simulink model "Direct"  (R2015b)
settings: Solver=VariableStepAuto  StartTime=0.0  StopTime=10.0  RelTol=1e-3
values from neighbouring files (symbols this model uses):
  f = 50    [DirectControl2.m]
  L = XL/(2*2*pi*f)    (= 0.159154943092)    [DirectControl2.m]
  Sbase = 1000e6/2    (= 500000000)    [DirectControl2.m]
  Ts = 5e-6    (= 5e-06)    [DirectControl2.m]
  Tsample = 5e-4    (= 0.0005)    [DirectControl2.m]
  Vdc = 5    [DirectControl2.m]
  Vr = 220e3    (= 220000)    [DirectControl2.m]
  Vs = 220e3    (= 220000)    [DirectControl2.m]
undefined symbols (not defined in the file or in its folder): Ki, Kp
libraries: powerlib_meascontrol x32, powerlib x28, simulink x2, simulink_extras x1
settings Model: Creator=Sourabh Suri  LastModifiedBy=Sourabh Suri

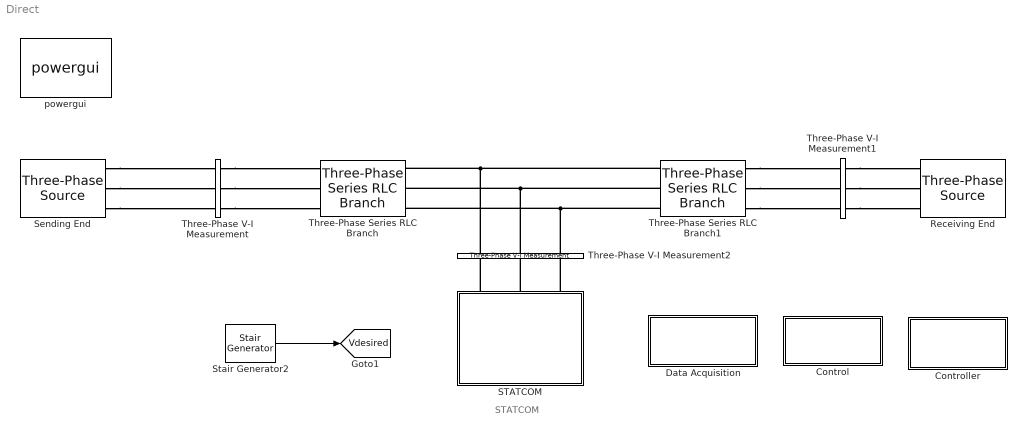
== system Direct ==
  note: STATCOM
  Control : Subsystem
  Controller : Subsystem
  Data Acquisition : Subsystem
  Receiving End : powerlib/Electrical Sources/Three-Phase Source  InternalConnection=Yg  VoltagePhases=off  Voltage=Vr  PhaseAngle=dr  Voltage_phases=[25e3 25e3 25e3]/sqrt(3)  PhaseAngles_phases=[0 -120 +120]  Frequency=f  NonIdealSource=off  SpecifyImpedance=off  Resistance=0.8929  Inductance=16.58e-3  ShortCircuitLevel=100e6  BaseVoltage=25e3  XRratio=7  BusType=swing  Pref=10e3  Qref=0  Prefabc=[10e3, 10e3, 10e3]  Qrefabc=[0, 0, 0]  Qmin=-inf  Qmax=inf
  STATCOM : Subsystem
  Sending End : powerlib/Electrical Sources/Three-Phase Source  InternalConnection=Yg  VoltagePhases=off  Voltage=Vs  PhaseAngle=ds  Voltage_phases=[25e3 25e3 25e3]/sqrt(3)  PhaseAngles_phases=[0 -120 +120]  Frequency=f  NonIdealSource=off  SpecifyImpedance=off  Resistance=0  Inductance=0  ShortCircuitLevel=100e6  BaseVoltage=0  XRratio=7  BusType=swing  Pref=10e3  Qref=0  Prefabc=[10e3, 10e3, 10e3]  Qrefabc=[0, 0, 0]  Qmin=-inf  Qmax=inf
  Stair Generator2 : powerlib_meascontrol/Pulse & Signal Generators/Stair Generator  t=[0 1 2 3 4 5 6 7]  e=[ 0.07 0.08 0.09 0.1 0.11 0.12 0.13 0.07]  Ts=Ts
  Three-Phase Series RLC Branch : powerlib/Elements/Three-Phase Series RLC Branch  LConnTagsString=A|B|C  RConnTagsString=A|B|C  BranchType=L  Resistance=1  Inductance=L  Capacitance=1e-6  Measurements=None
  Three-Phase Series RLC Branch1 : powerlib/Elements/Three-Phase Series RLC Branch  LConnTagsString=A|B|C  RConnTagsString=A|B|C  BranchType=L  Resistance=1  Inductance=L  Capacitance=1e-6  Measurements=None
  Three-Phase V-I Measurement : powerlib/Measurements/Three-Phase V-I Measurement  VoltageMeasurement=phase-to-phase  SetLabelV=on  LabelV=Vsabc  Vpu=off  VpuLL=on  CurrentMeasurement=yes  SetLabelI=on  LabelI=Isabc  Ipu=on  Pbase=Sbase  Vbase=Vn  OutputType=Complex  PhasorSimulation=off  PSBequivalent=0
  Three-Phase V-I Measurement1 : powerlib/Measurements/Three-Phase V-I Measurement  VoltageMeasurement=phase-to-phase  SetLabelV=on  LabelV=Vrabc  Vpu=off  VpuLL=on  CurrentMeasurement=yes  SetLabelI=on  LabelI=Irabc  Ipu=on  Pbase=Sbase  Vbase=Vn  OutputType=Complex  PhasorSimulation=off  PSBequivalent=0
  Three-Phase V-I Measurement2 : powerlib/Measurements/Three-Phase V-I Measurement  VoltageMeasurement=phase-to-phase  SetLabelV=on  LabelV=Vmabc  Vpu=off  VpuLL=on  CurrentMeasurement=yes  SetLabelI=on  LabelI=Imabc  Ipu=on  Pbase=Sbase  Vbase=Vn  OutputType=Complex  PhasorSimulation=off  PSBequivalent=0
  powergui : powerlib/powergui  Priority=1  SimulationMode=Discrete  SolverType=Backward Euler  SampleTime=Ts  frequency=60  SPID=on  DisableSnubberDevices=on  DisableRonSwitches=on  DisableVfSwitches=on  SwTol=0  DisplayEquations=off  Interpol=off  ExternalGateDelay=off  methode=off  Ts=10  FunctionMessages=off  echomessages=off  HookPort=off  EnableUseOfTLC=off  x0status=blocks  frequencyindice=50  Pbase=100e6  ErrMax=1e-4  Iterations=50  UnitsV=kV  UnitsW=MW  buscounter=0  RestoreLinks=warning  ResistiveCurrentMeasurement=off  Frange=[0:2:500]  Ylog=off  Xlog=on  ShowGrid=off  save=off  variable=ZData  structure=0  ZoomFFT=off  StartTime=0.0  cycles=1  DisplayStyle=1  fundamental=60  FreqAxis=off  MaxFrequency=1000  frequencyindicesteady=1  RmsSteady=1  display=off
  tag scope: Vdesired=global
  wires:
  Stair Generator2/1 -> [Vdesired]
  connections:
  Three-Phase V-I Measurement2/RConn1 -- Three-Phase Series RLC Branch/RConn1 -- Three-Phase Series RLC Branch1/RConn1
  Three-Phase V-I Measurement2/RConn2 -- Three-Phase Series RLC Branch/RConn2 -- Three-Phase Series RLC Branch1/RConn2
  Three-Phase V-I Measurement2/RConn3 -- Three-Phase Series RLC Branch/RConn3 -- Three-Phase Series RLC Branch1/RConn3
  Sending End/RConn1 -- Three-Phase V-I Measurement/LConn1
  Sending End/RConn2 -- Three-Phase V-I Measurement/LConn2
  Three-Phase V-I Measurement1/LConn2 -- Receiving End/RConn2
  Three-Phase V-I Measurement1/LConn1 -- Receiving End/RConn1
  Three-Phase Series RLC Branch1/LConn3 -- Three-Phase V-I Measurement1/RConn3
  Three-Phase V-I Measurement/RConn2 -- Three-Phase Series RLC Branch/LConn2
  Three-Phase V-I Measurement/RConn1 -- Three-Phase Series RLC Branch/LConn1
  Three-Phase V-I Measurement1/LConn3 -- Receiving End/RConn3
  Three-Phase V-I Measurement/RConn3 -- Three-Phase Series RLC Branch/LConn3
  Three-Phase Series RLC Branch1/LConn1 -- Three-Phase V-I Measurement1/RConn1
  Three-Phase Series RLC Branch1/LConn2 -- Three-Phase V-I Measurement1/RConn2
  Sending End/RConn3 -- Three-Phase V-I Measurement/LConn3
  STATCOM/LConn1 -- Three-Phase V-I Measurement2/LConn1
  STATCOM/LConn2 -- Three-Phase V-I Measurement2/LConn2
  STATCOM/LConn3 -- Three-Phase V-I Measurement2/LConn3

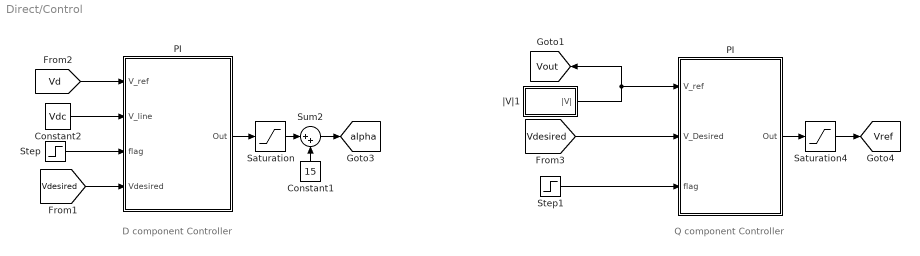
== system Direct/Control ==
  note: Q component Controller
  note: D component Controller
  Constant1 : Constant  Value=15
  Constant2 : Constant  Value=Vdc
  PI : MATLAB Function  TreatAsAtomicUnit=on
  "PI " : MATLAB Function  TreatAsAtomicUnit=on
  Saturation : Saturate  UpperLimit=45  LowerLimit=-25
  Saturation4 : Saturate  UpperLimit=1/sqrt(3)  LowerLimit=0.057
  Step : Step  Time=0.1  SampleTime=0
  Step1 : Step  Time=.04  SampleTime=0
  Sum2 : Sum  Inputs=|++  SaturateOnIntegerOverflow=on  InputSameDT=on  OutDataTypeStr=Inherit: Same as first input
  |V|1 : Subsystem
  tag scope: Vout=global, Vref=global, alpha=global
  wires:
  [Vd] -> PI/1(V_ref)
  PI/1(Out) -> Saturation/1
  Constant1/1 -> Sum2/2
  Step/1 -> PI/3(flag)
  Constant2/1 -> PI/2(V_line)
  |V|1/1(|V|) -> "PI "/1(V_ref), [Vout]
  "PI "/1(Out) -> Saturation4/1
  [Vdesired] -> "PI "/2(V_Desired)
  Step1/1 -> "PI "/3(flag)
  Saturation4/1 -> [Vref]
  Saturation/1 -> Sum2/1
  [Vdesired] -> PI/4(Vdesired)
  Sum2/1 -> [alpha]

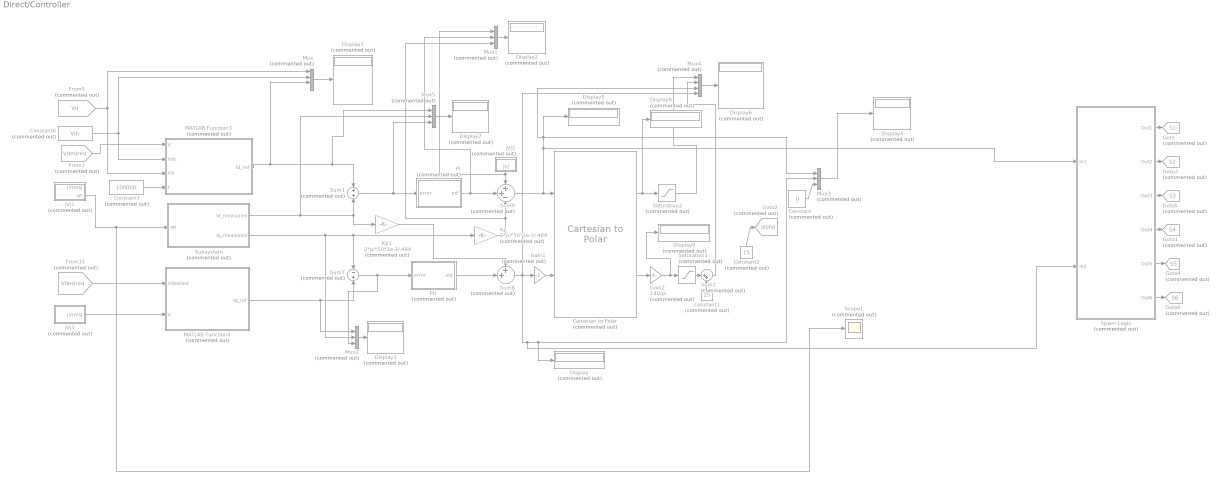
== system Direct/Controller ==
  Cartesian to Polar : simulink_extras/Transformations/Cartesian to Polar  Commented=on
  Constant : Constant  Commented=on  Value=0
  Constant1 : Constant  Commented=on  Value=15
  Constant2 : Constant  Commented=on  Value=15
  Constant3 : Constant  Commented=on  Value=100000
  Constant6 : Constant  Commented=on  Value=Vdc
  Display{,1..9} (10 alike) : Display  Commented=on
  From1 : From  Commented=on  GotoTag=Vdesired  TagVisibility=global
  From11 : From  Commented=on  GotoTag=Vdesired  TagVisibility=global
  From5 : From  Commented=on  GotoTag=Vd  TagVisibility=global
  Gain1 : Gain  Commented=on  Gain=-1
  Gain2 : Gain  Commented=on  Gain=180/pi
  Goto : Goto  Commented=on  GotoTag=S1  TagVisibility=global
  Goto1 : Goto  Commented=on  GotoTag=S4  TagVisibility=global
  Goto2 : Goto  Commented=on  GotoTag=alpha  TagVisibility=global
  Goto3 : Goto  Commented=on  GotoTag=S2  TagVisibility=global
  Goto4 : Goto  Commented=on  GotoTag=S5  TagVisibility=global
  Goto5 : Goto  Commented=on  GotoTag=S3  TagVisibility=global
  Goto6 : Goto  Commented=on  GotoTag=S6  TagVisibility=global
  Kp : Gain  Commented=on  Gain=2*pi*50*1e-3/.484
  Kp1 : Gain  Commented=on  Gain=2*pi*50*1e-3/.484
  MATLAB Function3 : MATLAB Function  Commented=on  TreatAsAtomicUnit=on
  MATLAB Function4 : MATLAB Function  Commented=on  TreatAsAtomicUnit=on
  Mux : Mux  Commented=on
  Mux{1..3,5} (4 alike) : Mux  Commented=on  Inputs=3
  Mux4 : Mux  Commented=on
  PI : Subsystem  Commented=on
  PI1 : Subsystem  Commented=on
  Saturation1 : Saturate  Commented=on  UpperLimit=2  LowerLimit=-28.5  LinearizeAsGain=off  ZeroCross=off
  Saturation2 : Saturate  Commented=on  UpperLimit=Vdc/sqrt(3)  LowerLimit=Vdc*.1e-9
  Scope1 : Scope  Commented=on
  Spwm Logic : Subsystem  Commented=on
  Subsystem : Subsystem  Commented=on
  Sum1 : Sum  Commented=on
  Sum2 : Sum  Commented=on  Inputs=|++  SaturateOnIntegerOverflow=on  InputSameDT=on  OutDataTypeStr=Inherit: Same as first input
  Sum7 : Sum  Commented=on  Inputs=-+
  Sum8 : Sum  Commented=on  Inputs=++|
  Sum9 : Sum  Commented=on  Inputs=++-
  |V|1 : Subsystem  Commented=on
  |V|2 : Subsystem  Commented=on
  |V|3 : Subsystem  Commented=on
  wires:
  Constant6/1 -> MATLAB Function3/2(Vdc), Mux/2
  From5/1 -> MATLAB Function3/3(Vd), Mux/1
  Mux/1 -> Display1/1
  |V|2/1(|V|) -> Mux1/1, Sum9/1
  Subsystem/2(Iq_measured) -> Mux2/2, Kp/1, Sum7/1
  Kp/1 -> Mux1/3, Sum9/3
  From11/1 -> MATLAB Function4/1(Vdesired)
  |V|3/1(|Vrms|) -> MATLAB Function4/2(V)
  Sum7/1 -> Mux2/3, PI1/1(error)
  PI1/1(eq') -> Sum8/2
  Kp1/1 -> Sum8/1
  Mux4/1 -> Display6/1
  Subsystem/1(Id_measured) -> Mux5/2, Kp1/1, Sum1/2
  MATLAB Function3/1(Id_ref) -> Mux5/1, Sum1/1, Mux/3
  Mux5/1 -> Display7/1
  Sum1/1 -> Mux5/3, PI/1(error)
  Cartesian to Polar/1 -> Display8/1, Saturation2/1
  Mux1/1 -> Display2/1
  PI/1(ed') -> Mux1/2, Sum9/2
  Mux2/1 -> Display3/1
  MATLAB Function4/1(Iq_ref) -> Mux2/1, Sum7/2
  Mux3/1 -> Display4/1
  |V|1/2(wt) -> Scope1/1, Subsystem/1(wt)
  Constant/1 -> Mux3/3
  Saturation1/1 -> Sum2/1
  Constant1/1 -> Sum2/2
  Sum8/1 -> Spwm Logic/2(In2), Display/1, Mux3/2, Gain1/1, Mux4/4
  Sum2/1 -> Mux4/2
  Saturation2/1 -> Mux4/1
  Cartesian to Polar/2 -> Gain2/1
  Gain1/1 -> Cartesian to Polar/2
  Sum9/1 -> Mux4/3, Mux3/1, Display5/1, Spwm Logic/1(In1), Cartesian to Polar/1
  Constant2/1 -> Goto2/1
  Spwm Logic/2(Out2) -> Goto3/1
  Spwm Logic/1(Out1) -> Goto/1
  Spwm Logic/3(Out3) -> Goto5/1
  Spwm Logic/4(Out4) -> Goto1/1
  Spwm Logic/5(Out5) -> Goto4/1
  Spwm Logic/6(Out6) -> Goto6/1
  Constant3/1 -> MATLAB Function3/4(t)
  From1/1 -> MATLAB Function3/1(V)
  Gain2/1 -> Display9/1, Saturation1/1

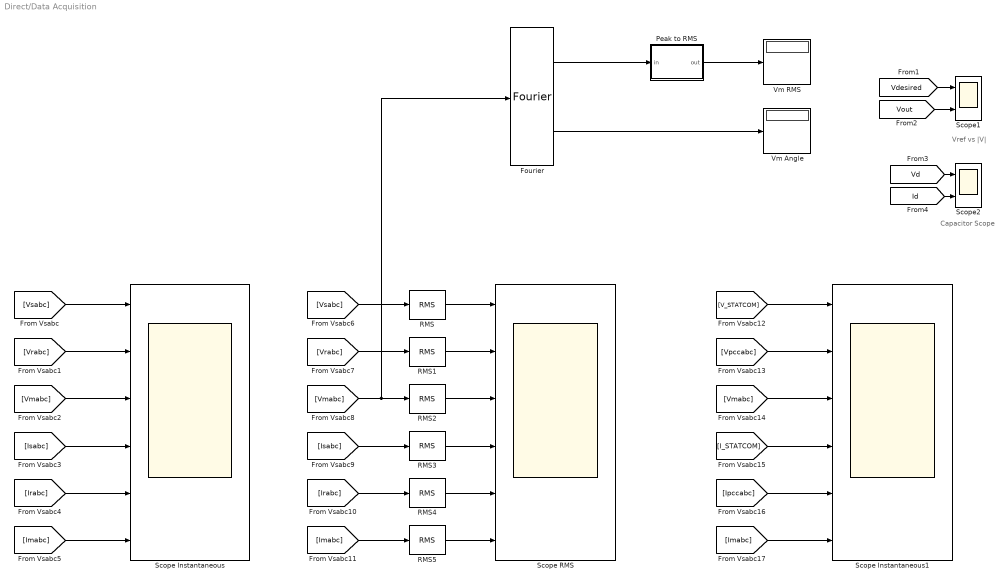
== system Direct/Data Acquisition ==
  note: Vref vs |V|
  note: Capacitor Scope
  Fourier : powerlib_meascontrol/Measurements/Fourier  Freq=f  n=1  InInit=[0, 0]  Ts=0
  Peak to RMS : MATLAB Function  TreatAsAtomicUnit=on
  RMS{,1..5} (6 alike) : powerlib_meascontrol/Measurements/RMS  TrueRMS=off  Freq=f  RMSInit=0  Ts=0
  Scope Instantaneous : Scope  NumInputPorts=6
  Scope Instantaneous1 : Scope  NumInputPorts=6
  Scope RMS : Scope  NumInputPorts=6
  Scope1 : Scope  NumInputPorts=2
  Scope2 : Scope  NumInputPorts=2
  Vm Angle : Display
      settings: Decimation=3
  Vm RMS : Display
      settings: Decimation=3
  wires:
  [Vsabc] -> Scope Instantaneous/1
  [Vrabc] -> Scope Instantaneous/2
  [Irabc] -> Scope Instantaneous/5
  [Imabc] -> Scope Instantaneous/6
  [Vmabc] -> Scope Instantaneous/3
  [Isabc] -> Scope Instantaneous/4
  RMS/1 -> Scope RMS/1
  [Vrabc] -> RMS1/1
  RMS1/1 -> Scope RMS/2
  [Vmabc] -> Fourier/1, RMS2/1
  [Isabc] -> RMS3/1
  RMS3/1 -> Scope RMS/4
  [Irabc] -> RMS4/1
  RMS4/1 -> Scope RMS/5
  [Imabc] -> RMS5/1
  RMS5/1 -> Scope RMS/6
  RMS2/1 -> Scope RMS/3
  Fourier/2 -> Vm Angle/1
  [Vsabc] -> RMS/1
  Peak to RMS/1(out) -> Vm RMS/1
  Fourier/1 -> Peak to RMS/1(in)
  [V_STATCOM] -> Scope Instantaneous1/1
  [Vpccabc] -> Scope Instantaneous1/2
  [Ipccabc] -> Scope Instantaneous1/5
  [Imabc] -> Scope Instantaneous1/6
  [Vmabc] -> Scope Instantaneous1/3
  [I_STATCOM] -> Scope Instantaneous1/4
  [Vdesired] -> Scope1/1
  [Vout] -> Scope1/2
  [Vd] -> Scope2/1
  [Id] -> Scope2/2
  ? -> ?

== system Direct/STATCOM ==
  Inverter : Subsystem
  SVM : Subsystem
  Three-Phase Transformer (Two Windings)2 : powerlib/Elements/Three-Phase Transformer (Two Windings)  Winding1Connection=Y  Winding2Connection=Yg  CoreType=Three-limb core (core-type)  SetSaturation=off  Hysteresis=off  DataFile='hysteresis'  SetInitialFlux=off  Measurements=None  UNITS=SI  NominalPower=[ Sbase*1000 , 50 ]  Winding1=[22e+04 1e-9 0 ]  Winding2=[22e+03 1e-9 0]  Rm=inf  Lm=inf  L0=0.5  Saturation=[0 0;4.3111 686.13;1796.3 869.1]  InitialFluxes=[457.42 -457.42 400.24]  MoreParameters=off  BreakLoop=off  DataType=on  TransfoNumber=1
  Three-Phase V-I Measurement1 : powerlib/Measurements/Three-Phase V-I Measurement  VoltageMeasurement=phase-to-phase  SetLabelV=on  LabelV=Vpccabc  Vpu=off  VpuLL=on  CurrentMeasurement=yes  SetLabelI=on  LabelI=Ipccabc  Ipu=on  Pbase=Sbase  Vbase=Vn  OutputType=Complex  PhasorSimulation=off  PSBequivalent=0
  Three-Phase V-I Measurement3 : powerlib/Measurements/Three-Phase V-I Measurement  VoltageMeasurement=phase-to-ground  SetLabelV=on  LabelV=Vpcc  Vpu=on  VpuLL=off  CurrentMeasurement=yes  SetLabelI=on  LabelI=Ipcc  Ipu=on  Pbase=Sbase  Vbase=Vn  OutputType=Complex  PhasorSimulation=off  PSBequivalent=0
  A : PMIOPort  Port=1  Side=Left
  B : PMIOPort  Port=2  Side=Left
  C : PMIOPort  Port=3  Side=Left
  connections:
  Three-Phase Transformer (Two Windings)2/LConn1 -- A/RConn1
  Three-Phase Transformer (Two Windings)2/LConn2 -- B/RConn1
  Three-Phase Transformer (Two Windings)2/LConn3 -- C/RConn1
  Inverter/LConn1 -- Three-Phase V-I Measurement1/LConn1
  Inverter/LConn2 -- Three-Phase V-I Measurement1/LConn2
  Inverter/LConn3 -- Three-Phase V-I Measurement1/LConn3
  Three-Phase V-I Measurement3/LConn1 -- Three-Phase V-I Measurement1/RConn1
  Three-Phase V-I Measurement3/LConn2 -- Three-Phase V-I Measurement1/RConn2
  Three-Phase V-I Measurement3/LConn3 -- Three-Phase V-I Measurement1/RConn3
  Three-Phase V-I Measurement3/RConn1 -- Three-Phase Transformer (Two Windings)2/RConn1
  Three-Phase V-I Measurement3/RConn3 -- Three-Phase Transformer (Two Windings)2/RConn3
  Three-Phase Transformer (Two Windings)2/RConn2 -- Three-Phase V-I Measurement3/RConn2

== system Direct/Control/|V|1 ==
  Demux2 : Demux  Outputs=3
  MATLAB Function3 : MATLAB Function  TreatAsAtomicUnit=on
  PLL (3ph)2 : powerlib_meascontrol/PLL/PLL (3ph)  Fmin=45  Par_Init=[3.7 50.1]  ParK=[60 1400 0]  TcD=1.6e-4  MaxRateChangeFreq=10  FilterCutOffFreq=25  Ts=Ts  AGC=on
  Scope1 : Scope
  Second-Order Low Pass Filter2 : powerlib_meascontrol/Filters/Second-Order Filter  FilterType=Bandpass  Fo=50  Zeta=.707  Ts=Ts  Initialize=off  Vac_Init="[0,  0,  60]"  Vdc_Init=0  PlotResponse=off  FreqRange=[0, 100, 1]
      settings: AttributesFormatString=f0: %<Fo>
  Second-Order Low Pass Filter3 : powerlib_meascontrol/Filters/Second-Order Filter  FilterType=Lowpass  Fo=50  Zeta=0.707  Ts=Ts  Initialize=off  Vac_Init="[0,  0,  60]"  Vdc_Init=0  PlotResponse=off  FreqRange=[0, 50, 1]
      settings: AttributesFormatString=f0: %<Fo>
  Terminator1 : Terminator
  Terminator2 : Terminator
  abc to dq2 : powerlib_meascontrol/Transformations/abc to dq0  Alignment=90 degrees behind phase A axis
  |V| : Outport
  wires:
  Second-Order Low Pass Filter3/1 -> |V|/1
  Demux2/2 -> MATLAB Function3/2(u2)
  abc to dq2/1 -> Demux2/1
  Demux2/1 -> MATLAB Function3/1(u1)
  MATLAB Function3/1(abs_V) -> Second-Order Low Pass Filter3/1
  PLL (3ph)2/2 -> abc to dq2/2
  Demux2/3 -> Terminator2/1
  PLL (3ph)2/1 -> Terminator1/1
  Second-Order Low Pass Filter2/1 -> PLL (3ph)2/1, Scope1/1, abc to dq2/1
  [Vpccabc] -> Second-Order Low Pass Filter2/1

== system Direct/Controller/PI ==
  error : Inport
  Integrator : Integrator  LimitOutput=on  IgnoreLimit=on
  Ki : Gain  Gain=Ki
  Kp : Gain  Gain=Kp
  Sum8 : Sum  Inputs=|++
  ed' : Outport
  wires:
  error/1 -> Ki/1, Kp/1
  Integrator/1 -> Sum8/2
  Sum8/1 -> ed'/1
  Kp/1 -> Sum8/1
  Ki/1 -> Integrator/1

== system Direct/Controller/PI1 ==
  error : Inport
  Integrator : Integrator  LimitOutput=on
  Ki : Gain  Gain=Ki
  Kp : Gain  Gain=Kp
  Sum8 : Sum  Inputs=|++
  eq' : Outport
  wires:
  Ki/1 -> Integrator/1
  Kp/1 -> Sum8/1
  Sum8/1 -> eq'/1
  Integrator/1 -> Sum8/2
  error/1 -> Kp/1, Ki/1

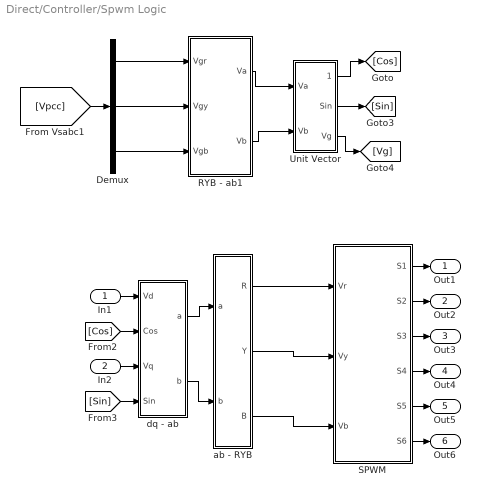
== system Direct/Controller/Spwm Logic ==
  In1 : Inport
  In2 : Inport  Port=2
  Demux : Demux  Outputs=3
  RYB - ab1 : Subsystem
  SPWM : Subsystem
  Unit Vector : Subsystem
  ab - RYB : Subsystem
  dq - ab : Subsystem
  Out1 : Outport
  Out2 : Outport  Port=2
  Out3 : Outport  Port=3
  Out4 : Outport  Port=4
  Out5 : Outport  Port=5
  Out6 : Outport  Port=6
  wires:
  SPWM/5(S5) -> Out5/1
  In2/1 -> dq - ab/3(Vq)
  SPWM/6(S6) -> Out6/1
  SPWM/2(S2) -> Out2/1
  In1/1 -> dq - ab/1(Vd)
  SPWM/3(S3) -> Out3/1
  SPWM/4(S4) -> Out4/1
  SPWM/1(S1) -> Out1/1
  [Sin] -> dq - ab/4(Sin)
  ab - RYB/1(R) -> SPWM/1(Vr)
  [Cos] -> dq - ab/2(Cos)
  dq - ab/2(b) -> ab - RYB/2(b)
  ab - RYB/2(Y) -> SPWM/2(Vy)
  ab - RYB/3(B) -> SPWM/3(Vb)
  dq - ab/1(a) -> ab - RYB/1(a)
  Demux/1 -> RYB - ab1/1(Vgr)
  Demux/3 -> RYB - ab1/3(Vgb)
  RYB - ab1/1(Va) -> Unit Vector/1(Va)
  Unit Vector/2(Sin) -> [Sin]
  Demux/2 -> RYB - ab1/2(Vgy)
  Unit Vector/1(Cos) -> [Cos]
  RYB - ab1/2(Vb) -> Unit Vector/2(Vb)
  Unit Vector/3(Vg) -> [Vg]
  [Vpcc] -> Demux/1

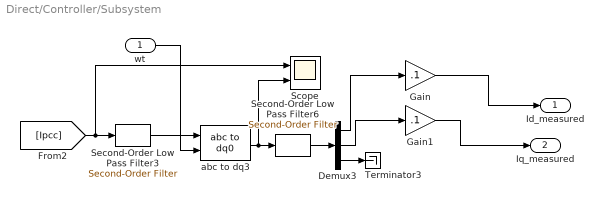
== system Direct/Controller/Subsystem ==
  wt : Inport
  Demux3 : Demux  Outputs=3
  Gain : Gain  Gain=.1
  Gain1 : Gain  Gain=.1
  Scope : Scope  NumInputPorts=2
  Second-Order Low Pass Filter3 : powerlib_meascontrol/Filters/Second-Order Filter  FilterType=Bandpass  Fo=50  Zeta=0.707  Ts=Ts  Initialize=off  Vac_Init="[0,  0,  60]"  Vdc_Init=0  PlotResponse=off  FreqRange=[0, 50, 1]
      settings: AttributesFormatString=f0: %<Fo>
  Second-Order Low Pass Filter6 : powerlib_meascontrol/Filters/Second-Order Filter  FilterType=Lowpass  Fo=25  Zeta=0.707  Ts=Ts  Initialize=off  Vac_Init="[0,  0,  60]"  Vdc_Init=0  PlotResponse=off  FreqRange=[0, 50, 1]
      settings: AttributesFormatString=f0: %<Fo>
  Terminator3 : Terminator
  abc to dq3 : powerlib_meascontrol/Transformations/abc to dq0  Alignment=90 degrees behind phase A axis
  Id_measured : Outport
  Iq_measured : Outport  Port=2
  wires:
  [Ipcc] -> Scope/1, Second-Order Low Pass Filter3/1
  Demux3/3 -> Terminator3/1
  Second-Order Low Pass Filter6/1 -> Demux3/1
  Demux3/1 -> Gain/1
  Demux3/2 -> Gain1/1
  Second-Order Low Pass Filter3/1 -> abc to dq3/1
  wt/1 -> abc to dq3/2
  abc to dq3/1 -> Scope/2, Second-Order Low Pass Filter6/1
  Gain/1 -> Id_measured/1
  Gain1/1 -> Iq_measured/1

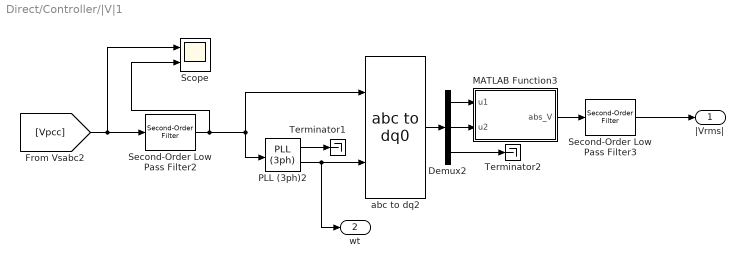
== system Direct/Controller/|V|1 ==
  Demux2 : Demux  Outputs=3
  MATLAB Function3 : MATLAB Function  TreatAsAtomicUnit=on
  PLL (3ph)2 : powerlib_meascontrol/PLL/PLL (3ph)  Fmin=45  Par_Init=[3.7 50.1]  ParK=[60 1400 0]  TcD=1.6e-4  MaxRateChangeFreq=10  FilterCutOffFreq=25  Ts=Ts  AGC=on
  Scope : Scope  NumInputPorts=2
  Second-Order Low Pass Filter2 : powerlib_meascontrol/Filters/Second-Order Filter  FilterType=Bandpass  Fo=50  Zeta=.707  Ts=Ts  Initialize=off  Vac_Init="[0,  0,  60]"  Vdc_Init=0  PlotResponse=off  FreqRange=[0, 100, 1]
      settings: AttributesFormatString=f0: %<Fo>
  Second-Order Low Pass Filter3 : powerlib_meascontrol/Filters/Second-Order Filter  FilterType=Lowpass  Fo=25  Zeta=0.707  Ts=Ts  Initialize=off  Vac_Init="[0,  0,  60]"  Vdc_Init=0  PlotResponse=off  FreqRange=[0, 50, 1]
      settings: AttributesFormatString=f0: %<Fo>
  Terminator1 : Terminator
  Terminator2 : Terminator
  abc to dq2 : powerlib_meascontrol/Transformations/abc to dq0  Alignment=90 degrees behind phase A axis
  |Vrms| : Outport
  wt : Outport  Port=2
  wires:
  Second-Order Low Pass Filter3/1 -> |Vrms|/1
  Demux2/2 -> MATLAB Function3/2(u2)
  abc to dq2/1 -> Demux2/1
  Demux2/1 -> MATLAB Function3/1(u1)
  MATLAB Function3/1(abs_V) -> Second-Order Low Pass Filter3/1
  PLL (3ph)2/2 -> wt/1, abc to dq2/2
  Demux2/3 -> Terminator2/1
  PLL (3ph)2/1 -> Terminator1/1
  [Vpcc] -> Scope/1, Second-Order Low Pass Filter2/1
  Second-Order Low Pass Filter2/1 -> PLL (3ph)2/1, abc to dq2/1, Scope/2

== system Direct/Controller/|V|2 ==
  Demux2 : Demux  Outputs=3
  MATLAB Function3 : MATLAB Function  TreatAsAtomicUnit=on
  PLL (3ph)2 : powerlib_meascontrol/PLL/PLL (3ph)  Fmin=45  Par_Init=[3.7 50.1]  ParK=[60 1400 0]  TcD=1.6e-4  MaxRateChangeFreq=10  FilterCutOffFreq=25  Ts=Ts  AGC=on
  Second-Order Low Pass Filter2 : powerlib_meascontrol/Filters/Second-Order Filter  FilterType=Bandpass  Fo=50  Zeta=.707  Ts=Ts  Initialize=off  Vac_Init="[0,  0,  60]"  Vdc_Init=0  PlotResponse=off  FreqRange=[0, 100, 1]
      settings: AttributesFormatString=f0: %<Fo>
  Second-Order Low Pass Filter3 : powerlib_meascontrol/Filters/Second-Order Filter  FilterType=Lowpass  Fo=50  Zeta=0.707  Ts=Ts  Initialize=off  Vac_Init="[0,  0,  60]"  Vdc_Init=0  PlotResponse=off  FreqRange=[0, 50, 1]
      settings: AttributesFormatString=f0: %<Fo>
  Terminator1 : Terminator
  Terminator2 : Terminator
  abc to dq2 : powerlib_meascontrol/Transformations/abc to dq0  Alignment=90 degrees behind phase A axis
  |V| : Outport
  wires:
  [Vpcc] -> Second-Order Low Pass Filter2/1
  Second-Order Low Pass Filter2/1 -> abc to dq2/1, PLL (3ph)2/1
  PLL (3ph)2/1 -> Terminator1/1
  Demux2/3 -> Terminator2/1
  PLL (3ph)2/2 -> abc to dq2/2
  MATLAB Function3/1(abs_V) -> Second-Order Low Pass Filter3/1
  Demux2/1 -> MATLAB Function3/1(u1)
  abc to dq2/1 -> Demux2/1
  Demux2/2 -> MATLAB Function3/2(u2)
  Second-Order Low Pass Filter3/1 -> |V|/1

== system Direct/Controller/|V|3 ==
  Demux2 : Demux  Outputs=3
  MATLAB Function3 : MATLAB Function  TreatAsAtomicUnit=on
  PLL (3ph)2 : powerlib_meascontrol/PLL/PLL (3ph)  Fmin=45  Par_Init=[3.7 50.1]  ParK=[60 1400 0]  TcD=1.6e-4  MaxRateChangeFreq=10  FilterCutOffFreq=25  Ts=Ts  AGC=on
  Scope1 : Scope
  Second-Order Low Pass Filter2 : powerlib_meascontrol/Filters/Second-Order Filter  FilterType=Bandpass  Fo=50  Zeta=.707  Ts=Ts  Initialize=off  Vac_Init="[0,  0,  60]"  Vdc_Init=0  PlotResponse=off  FreqRange=[0, 100, 1]
      settings: AttributesFormatString=f0: %<Fo>
  Second-Order Low Pass Filter3 : powerlib_meascontrol/Filters/Second-Order Filter  FilterType=Lowpass  Fo=50  Zeta=0.707  Ts=Ts  Initialize=off  Vac_Init="[0,  0,  60]"  Vdc_Init=0  PlotResponse=off  FreqRange=[0, 50, 1]
      settings: AttributesFormatString=f0: %<Fo>
  Terminator1 : Terminator
  Terminator2 : Terminator
  abc to dq2 : powerlib_meascontrol/Transformations/abc to dq0  Alignment=90 degrees behind phase A axis
  |Vrms| : Outport
  wires:
  Second-Order Low Pass Filter3/1 -> |Vrms|/1
  Demux2/2 -> MATLAB Function3/2(u2)
  abc to dq2/1 -> Demux2/1
  Demux2/1 -> MATLAB Function3/1(u1)
  MATLAB Function3/1(abs_V) -> Second-Order Low Pass Filter3/1
  PLL (3ph)2/2 -> abc to dq2/2
  Demux2/3 -> Terminator2/1
  PLL (3ph)2/1 -> Terminator1/1
  Second-Order Low Pass Filter2/1 -> PLL (3ph)2/1, Scope1/1, abc to dq2/1
  [Vpcc] -> Second-Order Low Pass Filter2/1

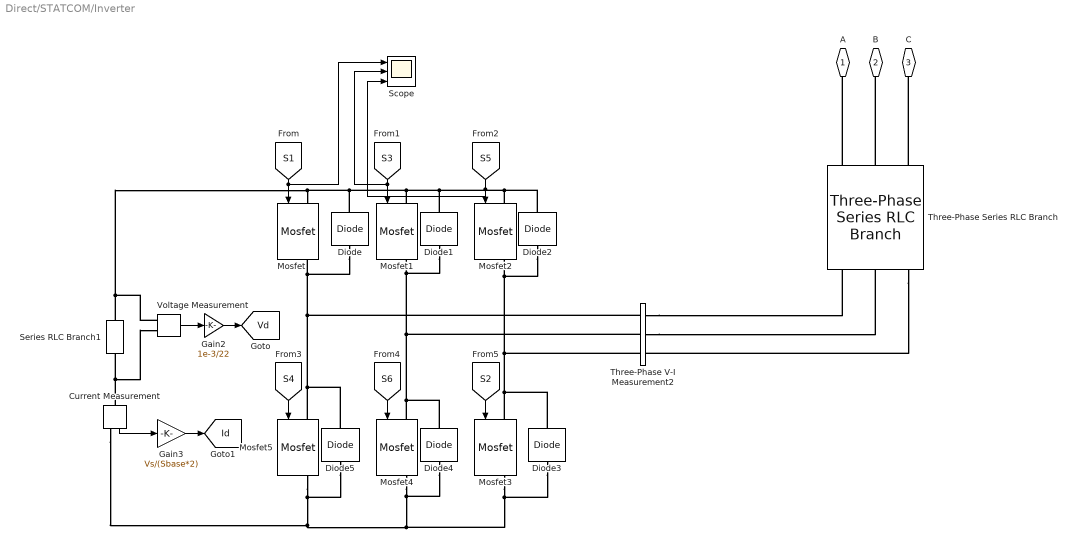
== system Direct/STATCOM/Inverter ==
  Current Measurement : powerlib/Measurements/Current Measurement  PhasorSimulation=off  OutputType=Complex  PSBequivalent=0
  Diode{,1..5} (6 alike) : powerlib/Power Electronics/Diode  Ron=0.001  Lon=0  Vf=0.8  IC=0  UseSnubber=off  Rs=inf  Cs=250e-9  Measurements=off
  Gain2 : Gain  Gain=1e-3/22
  Gain3 : Gain  Gain=Vs/(Sbase*2)
  Mosfet{,1..5} (6 alike) : powerlib/Power Electronics/Mosfet  Ron=0.1  Lon=0  Rd=0.01  Vfd=0  IC=0  Rs=1e5  Cs=inf  Measurements=on
  Scope : Scope  NumInputPorts=3
  Series RLC Branch1 : powerlib/Elements/Series RLC Branch  LConnTagsString=__new0  RConnTagsString=__new0  BranchType=C  Resistance=1  Inductance=1e-15  SetiL0=off  InitialCurrent=0  Capacitance=24e-4  Setx0=on  InitialVoltage=22e3*5  Measurements=None
  Three-Phase Series RLC Branch : powerlib/Elements/Three-Phase Series RLC Branch  LConnTagsString=A|B|C  RConnTagsString=A|B|C  BranchType=L  Resistance=.1  Inductance=1e-3  Capacitance=1e-6  Measurements=None
  Three-Phase V-I Measurement2 : powerlib/Measurements/Three-Phase V-I Measurement  VoltageMeasurement=phase-to-phase  SetLabelV=on  LabelV=V_STATCOM  Vpu=off  VpuLL=on  CurrentMeasurement=yes  SetLabelI=on  LabelI=I_STATCOM  Ipu=on  Pbase=Sbase  Vbase=Vn  OutputType=Complex  PhasorSimulation=off  PSBequivalent=0
  Voltage Measurement : powerlib/Measurements/Voltage Measurement  PhasorSimulation=off  OutputType=Complex  PSBequivalent=0
  A : PMIOPort  Port=1  Side=Left
  B : PMIOPort  Port=2  Side=Left
  C : PMIOPort  Port=3  Side=Left
  tag scope: Id=global, Vd=global
  wires:
  [S2] -> Mosfet3/1
  [S4] -> Mosfet5/1
  [S1] -> Scope/1, Mosfet/1
  [S5] -> Scope/3, Mosfet2/1
  [S6] -> Mosfet4/1
  Voltage Measurement/1 -> Gain2/1
  Current Measurement/1 -> Gain3/1
  Gain2/1 -> [Vd]
  Gain3/1 -> [Id]
  [S3] -> Scope/2, Mosfet1/1
  connections:
  Current Measurement/LConn1 -- Series RLC Branch1/RConn1 -- Voltage Measurement/LConn2
  Mosfet/RConn1 -- Three-Phase V-I Measurement2/LConn1 -- Diode5/RConn1 -- Mosfet5/LConn1 -- Diode/LConn1
  Mosfet1/RConn1 -- Three-Phase V-I Measurement2/LConn2 -- Diode4/RConn1 -- Mosfet4/LConn1 -- Diode1/LConn1
  Mosfet2/RConn1 -- Three-Phase V-I Measurement2/LConn3 -- Diode3/RConn1 -- Mosfet3/LConn1 -- Diode2/LConn1
  Three-Phase Series RLC Branch/LConn2 -- B/RConn1
  Three-Phase Series RLC Branch/LConn3 -- C/RConn1
  Three-Phase Series RLC Branch/LConn1 -- A/RConn1
  Three-Phase V-I Measurement2/RConn1 -- Three-Phase Series RLC Branch/RConn1
  Three-Phase V-I Measurement2/RConn2 -- Three-Phase Series RLC Branch/RConn2
  Three-Phase Series RLC Branch/RConn3 -- Three-Phase V-I Measurement2/RConn3
  Diode3/LConn1 -- Current Measurement/RConn1 -- Diode5/LConn1 -- Mosfet5/RConn1 -- Diode4/LConn1 -- Mosfet4/RConn1 -- Mosfet3/RConn1
  Voltage Measurement/LConn1 -- Mosfet/LConn1 -- Diode2/RConn1 -- Mosfet2/LConn1 -- Diode1/RConn1 -- Mosfet1/LConn1 -- Diode/RConn1 -- Series RLC Branch1/LConn1

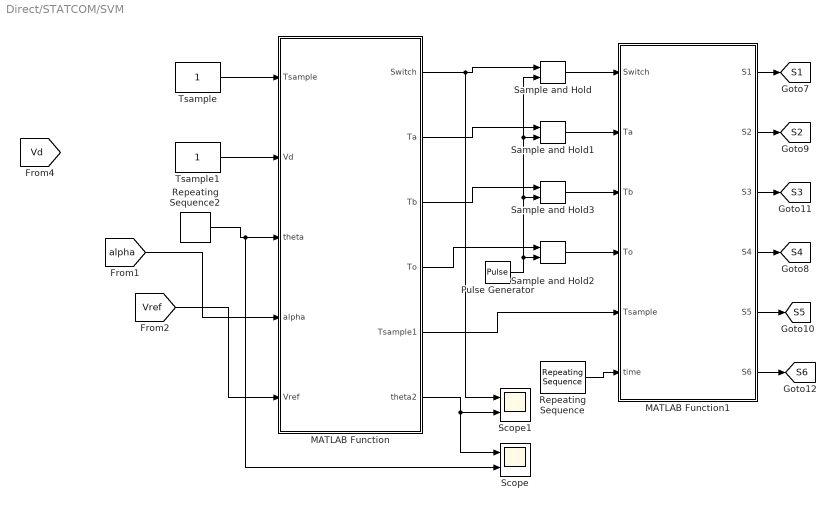
== system Direct/STATCOM/SVM ==
  MATLAB Function : MATLAB Function  TreatAsAtomicUnit=on
  MATLAB Function1 : MATLAB Function  TreatAsAtomicUnit=on
  Pulse Generator : DiscretePulseGenerator  PulseType=Time based  Period=Tsample  PulseWidth=0.1
  Repeating Sequence : simulink/Sources/Repeating Sequence  rep_seq_t=[0 Tsample ]  rep_seq_y=[0 1]
  Repeating Sequence2 : simulink/Sources/Repeating Sequence  rep_seq_t=[0 1/f ]  rep_seq_y=[0 (2*pi)]
  Sample and Hold{,1..3} (4 alike) : powerlib_meascontrol/Additional Components/Sample and Hold  ic=0  Ts=Tsample
  Scope : Scope  NumInputPorts=2
  Scope1 : Scope  NumInputPorts=2
  Tsample : Constant
  Tsample1 : Constant
  tag scope: S1=global, S2=global, S3=global, S4=global, S5=global, S6=global
  wires:
  MATLAB Function/1(Switch) -> Scope1/1, Sample and Hold/1
  Sample and Hold/1 -> MATLAB Function1/1(Switch)
  MATLAB Function/3(Tb) -> Sample and Hold3/1
  Sample and Hold1/1 -> MATLAB Function1/2(Ta)
  MATLAB Function/2(Ta) -> Sample and Hold1/1
  Sample and Hold2/1 -> MATLAB Function1/4(To)
  MATLAB Function/4(To) -> Sample and Hold2/1
  Pulse Generator/1 -> Sample and Hold/2, Sample and Hold1/2, Sample and Hold3/2, Sample and Hold2/2
  Tsample/1 -> MATLAB Function/1(Tsample)
  Repeating Sequence/1 -> MATLAB Function1/6(time)
  MATLAB Function/5(Tsample1) -> MATLAB Function1/5(Tsample)
  Sample and Hold3/1 -> MATLAB Function1/3(Tb)
  Repeating Sequence2/1 -> Scope/2, MATLAB Function/3(theta)
  [alpha] -> MATLAB Function/4(alpha)
  [Vref] -> MATLAB Function/5(Vref)
  MATLAB Function1/1(S1) -> [S1]
  MATLAB Function1/2(S2) -> [S2]
  MATLAB Function1/3(S3) -> [S3]
  MATLAB Function1/4(S4) -> [S4]
  MATLAB Function1/5(S5) -> [S5]
  MATLAB Function1/6(S6) -> [S6]
  MATLAB Function/6(theta2) -> Scope1/2, Scope/1
  Tsample1/1 -> MATLAB Function/2(Vd)

== system Direct/Controller/Spwm Logic/RYB - ab1 ==
  Vgr : Inport
  Vgy : Inport  Port=2
  Vgb : Inport  Port=3
  Demux : Demux  Outputs=2
  Gain : Gain  Gain=[1 -0.5 -0.5;0 0.866 -0.866]  Multiplication=Matrix(K*u)
  Mux : Mux  Inputs=3
  Scope : Scope  NumInputPorts=2
  Va : Outport
  Vb : Outport  Port=2
  wires:
  Demux/1 -> Va/1
  Mux/1 -> Scope/2, Gain/1
  Demux/2 -> Scope/1, Vb/1
  Vgr/1 -> Mux/1
  Vgb/1 -> Mux/3
  Gain/1 -> Demux/1
  Vgy/1 -> Mux/2

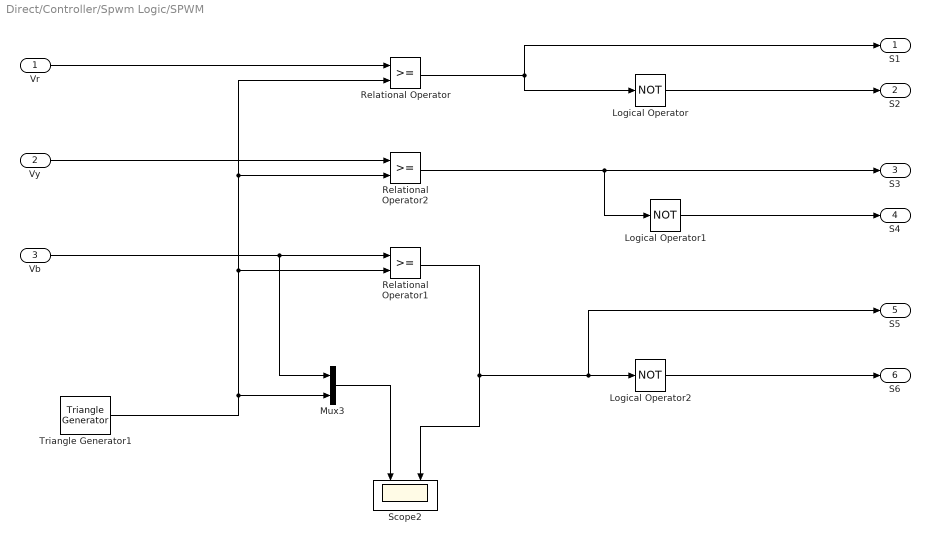
== system Direct/Controller/Spwm Logic/SPWM ==
  Vr : Inport
  Vy : Inport  Port=2
  Vb : Inport  Port=3
  Logical Operator : Logic  Operator=NOT  IconShape=distinctive  AllPortsSameDT=off  OutDataTypeStr=boolean
  Logical Operator1 : Logic  Operator=NOT  IconShape=distinctive  AllPortsSameDT=off  OutDataTypeStr=boolean
  Logical Operator2 : Logic  Operator=NOT  IconShape=distinctive  AllPortsSameDT=off  OutDataTypeStr=boolean
  Mux3 : Mux  Inputs=2
  Relational Operator : RelationalOperator  OutDataTypeStr=boolean
  Relational Operator1 : RelationalOperator  OutDataTypeStr=boolean
  Relational Operator2 : RelationalOperator  OutDataTypeStr=boolean
  Scope2 : Scope  NumInputPorts=2
  Triangle Generator1 : powerlib_meascontrol/Pulse & Signal Generators/Triangle Generator  Freq=5e3  Phase=90  Ts=Ts
  S1 : Outport
  S2 : Outport  Port=2
  S3 : Outport  Port=3
  S4 : Outport  Port=4
  S5 : Outport  Port=5
  S6 : Outport  Port=6
  wires:
  Triangle Generator1/1 -> Relational Operator2/2, Relational Operator/2, Relational Operator1/2, Mux3/2
  Relational Operator1/1 -> Scope2/2, S5/1, Logical Operator2/1
  Logical Operator1/1 -> S4/1
  Relational Operator/1 -> S1/1, Logical Operator/1
  Logical Operator2/1 -> S6/1
  Relational Operator2/1 -> Logical Operator1/1, S3/1
  Logical Operator/1 -> S2/1
  Mux3/1 -> Scope2/1
  Vb/1 -> Mux3/1, Relational Operator1/1
  Vy/1 -> Relational Operator2/1
  Vr/1 -> Relational Operator/1

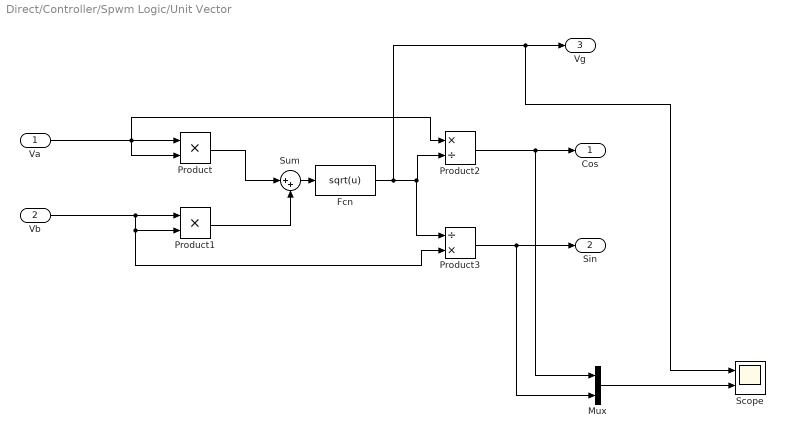
== system Direct/Controller/Spwm Logic/Unit Vector ==
  Va : Inport
  Vb : Inport  Port=2
  Fcn : Fcn  Expr=sqrt(u)
  Mux : Mux  Inputs=2
  Product : Product
  Product1 : Product
  Product2 : Product  Inputs=*/
  Product3 : Product  Inputs=/*
  Scope : Scope  NumInputPorts=2
  Sum : Sum  Inputs=|++
  Cos : Outport
  Sin : Outport  Port=2
  Vg : Outport  Port=3
  wires:
  Sum/1 -> Fcn/1
  Va/1 -> Product2/1, Product/2, Product/1
  Vb/1 -> Product1/1, Product1/2, Product3/2
  Product/1 -> Sum/1
  Product1/1 -> Sum/2
  Product3/1 -> Mux/2, Sin/1
  Product2/1 -> Mux/1, Cos/1
  Fcn/1 -> Scope/1, Vg/1, Product3/1, Product2/2
  Mux/1 -> Scope/2

== system Direct/Controller/Spwm Logic/ab - RYB ==
  a : Inport
  b : Inport  Port=2
  Demux : Demux  Outputs=3
  Gain : Gain  Gain=[1 0;-1/2 sqrt(3)/2;-1/2 -sqrt(3)/2]  Multiplication=Matrix(K*u)
  Mux : Mux  Inputs=2
  R : Outport
  Y : Outport  Port=2
  B : Outport  Port=3
  wires:
  b/1 -> Mux/2
  Gain/1 -> Demux/1
  a/1 -> Mux/1
  Demux/2 -> Y/1
  Mux/1 -> Gain/1
  Demux/1 -> R/1
  Demux/3 -> B/1

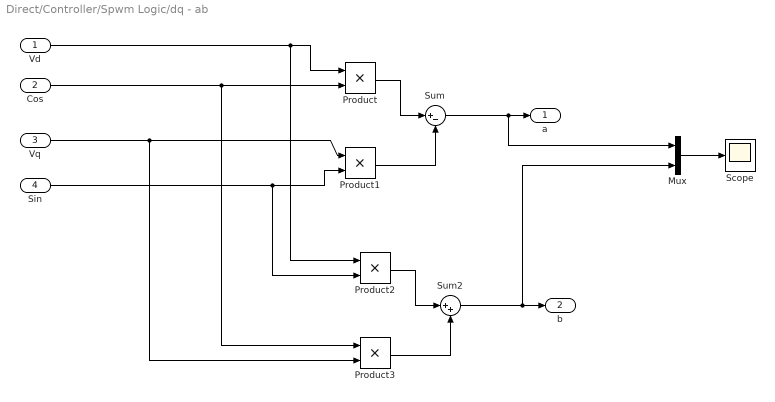
== system Direct/Controller/Spwm Logic/dq - ab ==
  Vd : Inport
  Cos : Inport  Port=2
  Vq : Inport  Port=3
  Sin : Inport  Port=4
  Mux : Mux  Inputs=2
  Product{,1..3} (4 alike) : Product
  Scope : Scope
  Sum : Sum  Inputs=|+-
  Sum2 : Sum  Inputs=|++
  a : Outport
  b : Outport  Port=2
  wires:
  Cos/1 -> Product/2, Product3/1
  Sum2/1 -> Mux/2, b/1
  Product3/1 -> Sum2/2
  Product2/1 -> Sum2/1
  Vq/1 -> Product1/1, Product3/2
  Sum/1 -> Mux/1, a/1
  Vd/1 -> Product/1, Product2/1
  Product1/1 -> Sum/2
  Sin/1 -> Product1/2, Product2/2
  Product/1 -> Sum/1
  Mux/1 -> Scope/1

== matlab function Direct/Data Acquisition/Peak to RMS ==
  data: in input; out output
function out = fcn(in)
% converts peak values to RMS values

out = in/sqrt(2);

== matlab function Direct/Control/PI  ==
  data: V_ref input; Out output; V_Desired input; flag input
function Out   = fcn(V_ref,V_Desired,flag)
%V_line=V_line/3;
integrator=0;
differential=0;
error=0;
% Kp=.0055;
% Ki=5e-5;
% Kd=0;
%  Kp=.0055;
%  Ki=0.0025;
% Kd=0;
  Kp=0.200;
 Ki=0.0007;
Kd=0;


persistent error_old;
if(isempty(error_old))
    error_old=0;
end 
 
persistent Vi;
if(isempty(Vi))
    Vi=0;
end
persistent Vref;

if(isempty(Vref))
    Vref=0;
end


 if flag==1
error=V_ref-V_Desired;
 
Vi=Vi+error;
differential= error - error_old;
integrator = Vi;
 end
 Out=-1*(Kp*error+Ki*integrator-Kd*differential);
 error_old = error;

== matlab function Direct/STATCOM/SVM/MATLAB Function ==
  data: Switch output; Ta output; Tb output; To output; Tsample1 output; Tsample input; Vd input; theta input; alpha input; Vref input; theta2 output
function [Switch, Ta, Tb, To, Tsample1,theta2]= fcn(Tsample,Vd, theta, alpha,Vref)
%#codegen
Tsample1 = Tsample;
%magnitude = abs(Vref*cosine+Vref*1i* sine);
%Vref= Vd*0.5;
Ta=0; Tb=0; To=0; %Tsample= 250e-6;

theta= theta+ 3*pi/2+(pi/90)+alpha*(pi/180);
Sector=1;

Switch = zeros(7,3);

if  theta>2*pi
    theta = -2*pi + theta;
end
if  theta<0
    theta = pi + theta;
end
theta2= theta;
if 0<theta && theta<=pi/3
    Sector= 1;
    
elseif pi/3<theta && theta<=2*pi/3
    Sector= 2;
    
elseif 2*pi/3<theta && theta<=pi
    Sector= 3;
    
elseif pi<theta && theta<=4*pi/3
    Sector= 4;
  
elseif 4*pi/3<theta && theta<=5*pi/3
    Sector= 5;
  
elseif 5*pi/3<theta && theta<=2*pi
    Sector= 6;

end


switch Sector
    case 1
     Ta = sqrt(3)* Tsample * Vref *sin((pi/3) - theta) / Vd;
     Tb = sqrt(3)* Tsample * Vref *sin(theta) / Vd;
     %To = Tsample - Ta - Tb;
     % Such that To/4, Ta/2, Tb/2, T0/2, Tb/2, Ta/2, To/2.
     % Here switching frequency will be sampling frequency
     % Van, Vbn, Vcn will be switched according to below sequence, 
     % 000, 100, 110, 111, 110, 100, 000.
     Switch = [0 0 0; 1 0 0; 1 1 0; 1 1 1; 1 1 0; 1 0 0; 0 0 0];
     
    case 2
     theta1 = theta - (pi/3);
     Ta = sqrt(3)* Tsample * Vref *sin((pi/3) - theta1) / Vd;
     Tb = sqrt(3)* Tsample * Vref *sin(theta1) / Vd;
     %To = Tsample - Ta - Tb;
     Switch = [0 0 0; 1 1 0; 0 1 0; 1 1 1; 0 1 0; 1 1 0; 0 0 0];
     
    case 3
     theta1 = theta - (2*pi/3);
     Ta = sqrt(3)* Tsample * Vref *sin((pi/3) - theta1) / Vd;
     Tb = sqrt(3)* Tsample * Vref *sin(theta1) / Vd;
     %To = Tsample - Ta - Tb;
     Switch = [0 0 0; 0 1 0; 0 1 1; 1 1 1; 0 1 1 ;0 1 0 ; 0 0 0];
     
    case 4
     theta1 = theta - (pi);
     Ta = sqrt(3)* Tsample * Vref *sin((pi/3) - theta1) / Vd;
     Tb = sqrt(3)* Tsample * Vref *sin(theta1) / Vd;
     %To = Tsample - Ta - Tb;
     Switch = [0 0 0;0 1 1; 0 0 1; 1 1 1; 0 0 1; 0 1 1; 0 0 0];
     
    case 5
     theta1 = theta - (4*pi/3);
     Ta = sqrt(3)* Tsample * Vref *sin((pi/3) - theta1) / Vd;
     Tb = sqrt(3)* Tsample * Vref *sin(theta1) / Vd;
     %To = Tsample - Ta - Tb;
     Switch = [0 0 0; 0 0 1; 1 0 1; 1 1 1; 1 0 1; 0 0 1; 0 0 0];
     
    case 6
     theta1 = theta - (5*pi/3);
     Ta = sqrt(3)* Tsample * Vref *sin((pi/3) - theta1) / Vd;
     Tb = sqrt(3)* Tsample * Vref *sin(theta1) / Vd;
     %To = Tsample - Ta - Tb;
     Switch = [0 0 0; 1 0 1; 1 0 0; 1 1 1; 1 0 0; 1 0 1; 0 0 0];
     
    otherwise
        Ta=0; Tb=0; To=0;
        
end
To = Tsample - Ta - Tb;

== matlab function Direct/STATCOM/SVM/MATLAB Function1 ==
  data: Switch input; Ta input; Tb input; To input; Tsample input; S1 output; S2 output; S3 output; time input; S4 output; S5 output; S6 output
function [S1, S2, S3, S4, S5, S6] = fcn(Switch, Ta, Tb, To, Tsample,time)
%#codegen  To/4, Ta/2, Tb/2, T0/2, Tb/2, Ta/2, To/2.
%Tsample= 250e-6;
S1=0;
S2=0;
S3=0;
S4=0;
S5=0;
S6=0;
% if time1 > Tsample
%     time1 = 0;
% end
% time= time1+ t;
if (0< time) && (time<= To/4)
    S1 = Switch(1,1);
    S2 = Switch(1,2);
    S3 = Switch(1,3);
elseif (To/4 < time) && (time <= To/4 +  Ta/2)
    S1 = Switch(2,1);
    S2 = Switch(2,2);
    S3 = Switch(2,3);   
elseif (To/4 +  Ta/2 < time) && (time <  To/4 +  Ta/2 + Tb/2)
    S1 = Switch(3,1);
    S2 = Switch(3,2);
    S3 = Switch(3,3); 
elseif (To/4 +  Ta/2 + Tb/2  < time) && (time <  To/4 +  Ta/2 + Tb/2 + To/2)
    S1 = Switch(4,1);
    S2 = Switch(4,2);
    S3 = Switch(4,3); 
elseif (To/4 +  Ta/2 + Tb/2 + To/2 < time) && (time <  To/4 +  Ta/2 + Tb/2 + To/2 + Tb/2)
    S1 = Switch(5,1);
    S2 = Switch(5,2);
    S3 = Switch(5,3);
elseif (To/4 +  Ta/2 + Tb/2 + To/2 + Tb/2 < time) && (time < To/4 +  Ta/2 + Tb/2 + To/2 + Tb/2 + Ta/2)
    S1 = Switch(6,1);
    S2 = Switch(6,2);
    S3 = Switch(6,3);
elseif (To/4 +  Ta/2 + Tb/2 + To/2 + Tb/2 + Ta/2 < time) && (time <  To/4 +  Ta/2 + Tb/2 + To/2 + Tb/2 + Ta/2 + To/4)
    S1 = Switch(7,1);
    S2 = Switch(7,2);
    S3 = Switch(7,3);
end
S1=S1;
S4= 1-S1;
S5=S3;
S3=S2;
S2= 1-S5;
S6= 1-S3;

== matlab function Direct/Control/PI ==
  data: V_ref input; Out output; V_line input; flag input; Vdesired input
function Out   = fcn(V_ref,V_line,flag,Vdesired)
%V_line=V_line/3;
error=0;
integrator=0;
differential=0;
%  Kp=0.50;
% Ki=.0003;
% Kd=0;
% Kp=120*(k);
% Ki=0.00005;
% Kd=0;
persistent error_old;
if(isempty(error_old))
    error_old=0;
end 
 
persistent Vi;
if(isempty(Vi))
    Vi=0;
end
persistent Vref;

if(isempty(Vref))
    Vref=0;
end

if(Vref~=Vdesired)
    Vi=0; error=0;
    integrator=0;
    differential=0;
    Vref=Vdesired;
end

       a =   2.426e-13;% (-4.613e-12, 5.098e-12)
       b =      -10.91;%  (-18.43, -3.398)
       c =     0.02122;%  (-0.08952, 0.132)
       k =     a*Vdesired^b+c;
       Kp=120*(k);
       Ki=0.00005;
       Kd=0;
if flag==1 
error=V_ref-V_line;

Vi=Vi+error;
differential= error - error_old;
integrator=Vi;
end 
 Out=(Kp*error+Ki*Vi+Kd*differential);
 error_old = error;
 Vrefout= Vref;

== matlab function Direct/Control/|V|1/MATLAB Function3 ==
  data: u1 input; u2 input; abs_V output
function abs_V = fcn(u1,u2)
%#codegen
abs_V= sqrt((u1*u1+u2*u2)/2);

== matlab function Direct/Controller/|V|1/MATLAB Function3 ==
  data: u1 input; u2 input; abs_V output
function abs_V = fcn(u1,u2)
%#codegen
abs_V= sqrt((u1*u1+u2*u2)/2);

== matlab function Direct/Controller/MATLAB Function3 ==
  data: V input; Vdc input; Id_ref output; Vd input; t input
function Id_ref  = fcn(V,Vdc,Vd,t)
Vbase_S = 220e3/sqrt(2); % Actual Base Value = 220KV. Scaling done to adjust woth matlab scaling
Sbase = 1000e6/2; % Actual Base Value = 1000MVA. Scaling done to adjust with matlab scaling
Ibase_S = Sbase/Vbase_S;
% V = V * Vbase_S;
% Vdc = Vdc * Vbase_S;
% Vd = Vd* Vbase_S;
C = (24e-4)*.484;
T = (V/Vdc)*(3/sqrt(2));
Gc= C/(t*T);
% Id_ref = Gc*(Vd - Vdc)/Ibase_S;
Id_ref = Gc*(Vd - Vdc);

== matlab function Direct/Controller/|V|2/MATLAB Function3 ==
  data: u1 input; u2 input; abs_V output
function abs_V = fcn(u1,u2)
%#codegen
abs_V= sqrt((u1*u1+u2*u2));

== matlab function Direct/Controller/|V|3/MATLAB Function3 ==
  data: u1 input; u2 input; abs_V output
function abs_V = fcn(u1,u2)
%#codegen
abs_V= sqrt((u1*u1+u2*u2)/2);

== matlab function Direct/Controller/MATLAB Function4 ==
  data: Vdesired input; Iq_ref output; V input
function Iq_ref = fcn(Vdesired,V)
% %#codegen
Iq_ref = (4/3)*sqrt(2)*(cosd(15)*Vdesired-Vdesired^2)/(V*(50/48.4));
